simulink model "iq"  (R2018a)
settings: Solver=FixedStepDiscrete  StartTime=0.0  StopTime=1e-2  RelTol=1e-3
libraries: simrfV2util1 x4, simrfV2systems x1
settings Model: Creator=Владимир  LastModifiedBy=Владимир

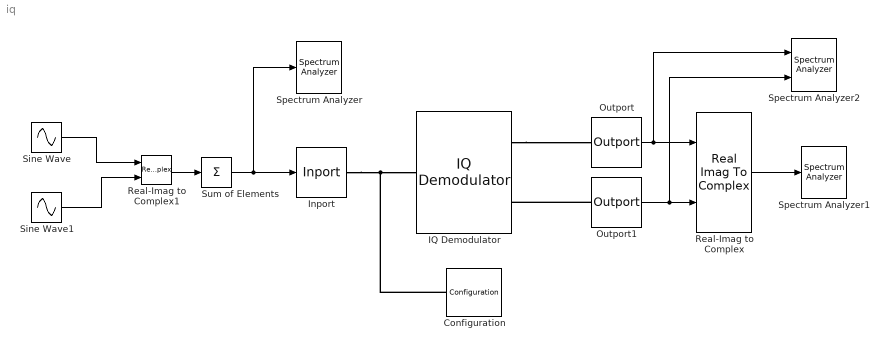
== system iq ==
  Configuration : simrfV2util1/Configuration  AutoFreq=on  Tones=[0] Hz  Harmonics=[1]  NormalizeCarrierPower=on  SolverType=Auto  UseCCode=on  StepSize=1e-8 s  AddNoise=on  defaultRNG=on  Seed=0  Temperature=290.0 K  SolverDelFlag=0  AbsTol=1e-6  RelTol=1e-3  MaxIter=10  ErrorEstimationType=2-norm over all variables
      settings: SourceProductName=RF Blockset  SourceProductBaseCode=RB
  IQ Demodulator : simrfV2systems/IQ Demodulator  classname=iqdemod  Source_linear_gain=Available power gain  linear_gain=10 dB  Poly_Coeffs=[0 1]  LOFreq=2 GHz  Zin=50  Zout=50  AddIRFilter=off  AddCSFilters=off  InternalGrounding=on  ForceNextInit=off  Source_Poly=Even and odd order  IPType=Output  IP2=inf dBm  IP3=20 dBm  P1dB=inf dBm  Psat=inf dBm  Gcomp=inf dBm  NF=6  GainMismatch=0.1 dB  PhaseMismatch=0 deg  Isolation=90 dB  AddPhaseNoise=off  PhaseNoiseOffset=1  PhaseNoiseLevel=-Inf  AutoImpulseLengthPN=on  ImpulseLengthPN=1e-10  ImpulseLength_unitPN=s  DesignMethodIR=Ideal  ResponseTypeIR=Highpass  ImplementationIR=LC Tee  ImplementationIdealIR=Constant per carrier  UseFilterOrderIR=on  FilterOrderIR=3  PassFreq_lpIR=1  PassFreq_lp_unitIR=GHz  PassFreq_hpIR=2  PassFreq_hp_unitIR=GHz  PassFreq_bpIR=[2 3]  PassFreq_bp_unitIR=GHz  PassFreq_bsIR=[1 4]  PassFreq_bs_unitIR=GHz  PassAttenIR=10*log10(2)  StopFreq_lpIR=2  StopFreq_lp_unitIR=GHz  StopFreq_hpIR=1  StopFreq_hp_unitIR=GHz  StopFreq_bpIR=[1.5 3.5]  StopFreq_bp_unitIR=GHz  StopFreq_bsIR=[2.1 2.9]  StopFreq_bs_unitIR=GHz  StopAttenIR=40  RsrcIR=50  RloadIR=50  AutoImpulseLengthIR=on  ImpulseLengthIR=1e-10  ImpulseLength_unitIR=s  DesignMethodCS=Ideal  ResponseTypeCS=Lowpass  ImplementationCS=LC Tee  ImplementationIdealCS=Constant per carrier  UseFilterOrderCS=on  FilterOrderCS=3  PassFreq_lpCS=1  PassFreq_lp_unitCS=GHz  PassFreq_hpCS=2  PassFreq_hp_unitCS=GHz  PassFreq_bpCS=[2 3]  PassFreq_bp_unitCS=GHz  PassFreq_bsCS=[1 4]  PassFreq_bs_unitCS=GHz  PassAttenCS=10*log10(2)  StopFreq_lpCS=2  StopFreq_lp_unitCS=GHz  StopFreq_hpCS=1  StopFreq_hp_unitCS=GHz  StopFreq_bpCS=[1.5 3.5]  StopFreq_bp_unitCS=GHz  StopFreq_bsCS=[2.1 2.9]  StopFreq_bs_unitCS=GHz  StopAttenCS=40  RsrcCS=50  RloadCS=50  AutoImpulseLengthCS=on  ImpulseLengthCS=1e-10  ImpulseLength_unitCS=s
      settings: SourceProductName=RF Blockset  SourceProductBaseCode=RB
  Inport : simrfV2util1/Inport  SimulinkInputSignalType=Power  CarrierFreq=2 GHz  ZS=50  InternalGrounding=on
      settings: SourceProductName=RF Blockset  SourceProductBaseCode=RB
  Outport : simrfV2util1/Outport  SensorType=Power  OutputFormat=Real Passband  CarrierFreq=0 GHz  ZL=50  InternalGrounding=on  StepSize=-1 s  AutoStep=off
      settings: SourceProductName=RF Blockset  SourceProductBaseCode=RB
  Outport1 : simrfV2util1/Outport  SensorType=Power  OutputFormat=Real Passband  CarrierFreq=0 GHz  ZL=50  InternalGrounding=on  StepSize=-1 s  AutoStep=off
      settings: SourceProductName=RF Blockset  SourceProductBaseCode=RB
  Real-Imag to Complex : RealImagToComplex
  Real-Imag to Complex1 : RealImagToComplex
  Sine Wave : Sin  Amplitude=1e-3  Frequency=[10e6 15e6]*2*pi  Phase=pi/2  SampleTime=1e-8
  Sine Wave1 : Sin  Amplitude=1e-3  Frequency=[10e6 15e6]*2*pi  SampleTime=1e-8
  Spectrum Analyzer : SpectrumAnalyzer
  Spectrum Analyzer1 : SpectrumAnalyzer
  Spectrum Analyzer2 : SpectrumAnalyzer  NumInputPorts=2
  Sum of Elements : Sum  Inputs=+
  wires:
  Sine Wave/1 -> Real-Imag to Complex1/1
  Sine Wave1/1 -> Real-Imag to Complex1/2
  Sum of Elements/1 -> Inport/1, Spectrum Analyzer/1
  Outport/1 -> Spectrum Analyzer2/1, Real-Imag to Complex/1
  Real-Imag to Complex/1 -> Spectrum Analyzer1/1
  Outport1/1 -> Spectrum Analyzer2/2, Real-Imag to Complex/2
  Real-Imag to Complex1/1 -> Sum of Elements/1
  connections:
  Inport/RConn1 -- Configuration/LConn1 -- IQ Demodulator/LConn1
  IQ Demodulator/RConn1 -- Outport/LConn1
  Outport1/LConn1 -- IQ Demodulator/RConn2
